simulink model "stateEstimator"  (R2021a)
settings: Solver=ode3  StartTime=0  StopTime=TFinal  FixedStep=Ts  RelTol=1e-3  EnableMultiTasking=on
undefined symbols (not defined in the file): DiscIntNeverNeededParam, Discrete, Estimator, g, init, Sensors, Time, Ts
libraries: simulink x27, ctrlSharedLib x3, sharedtransform x3, sharedutil x1
settings Model: Creator=The MathWorks, Inc.  LastModifiedBy=John
settings SolverCC: AlgebraicLoopSolver=TrustRegion
settings DataIOCC: LimitDataPoints=on  SaveFormat=Array  ReturnWorkspaceOutputs=off
settings OptimizationCC: BlockReduction=off  DefaultParameterBehavior=Inlined  BufferReuse=off  PassReuseOutputArgsThreshold=0
settings DebuggingCC: AlgebraicLoopMsg=none  ParameterPrecisionLossMsg=none  ParameterTunabilityLossMsg=error  UnconnectedInputMsg=none  UnconnectedOutputMsg=none  UnconnectedLineMsg=none  BusObjectLabelMismatch=error  SFUnexpectedBacktrackingDiag=warning  SFNoUnconditionalDefaultTransitionDiag=warning  SFExecutionAtInitializationDiag=none  SFMachineParentedDataDiag=warning  ArithmeticOperatorsInVariantConditions=warning
settings HardwareCC: ProdBitPerPointer=32  ProdBitPerSizeT=32  ProdBitPerPtrDiffT=32  ProdLargestAtomicInteger=Long  ProdWordSize=32  ProdHWDeviceType=ARM Compatible->ARM 9
settings ModelReferenceCC: ModelReferenceNumInstancesAllowed=Single  PropagateSignalLabelsOutOfModel=off
settings SFSimCC: SimUseLocalCustomCode=off  CustomCodeUndefinedFunction=UseInterfaceOnly
settings RTWCC: Description=Generic Real-Time Target  GenCodeOnly=on  GenerateReport=on  RTWUseLocalCustomCode=off  LaunchReport=on
settings CodeAppCC: ForceParamTrailComments=on  MaxIdLength=63  OperatorAnnotations=on  StateflowObjectComments=on  MATLABSourceComments=on
settings GRTTargetCC: TargetLangStandard=C89/C90 (ANSI)
settings ConfigComp: CovMetricSettings=dw  CovSaveCumulativeToWorkspaceVar=on  CovSaveSingleToWorkspaceVar=on  CovExternalEMLEnable=off  CovSFcnEnable=off

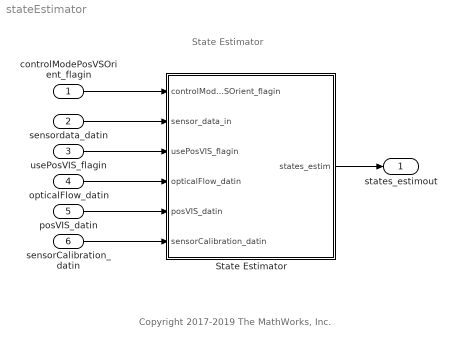
== system stateEstimator ==
  note: State Estimator
  note: Copyright 2017-2019 The MathWorks, Inc.
  controlModePosVSOrient_flagin : Inport  OutDataTypeStr=boolean  SampleTime=Ts
  sensordata_datin : Inport  Port=2  OutDataTypeStr=Bus: sensordata_t  SampleTime=Ts  BusOutputAsStruct=on
  usePosVIS_flagin : Inport  Port=3  OutDataTypeStr=single  SampleTime=Ts
  opticalFlow_datin : Inport  Port=4  OutDataTypeStr=single  SampleTime=Ts
  posVIS_datin : Inport  Port=5  OutDataTypeStr=single  SampleTime=Ts
  sensorCalibration_datin : Inport  Port=6  OutDataTypeStr=single  SampleTime=Ts
  State Estimator : Subsystem
  states_estimout : Outport  OutDataTypeStr=Bus: statesEstim_t  VectorParamsAs1DForOutWhenUnconnected=off  BusOutputAsStruct=on
  wires:
  State Estimator/1(states_estim) -> states_estimout/1
  opticalFlow_datin/1 -> State Estimator/4(opticalFlow_datin)
  controlModePosVSOrient_flagin/1 -> State Estimator/1(controlModePosVSOrient_flagin)
  usePosVIS_flagin/1 -> State Estimator/3(usePosVIS_flagin)
  posVIS_datin/1 -> State Estimator/5(posVIS_datin)
  sensordata_datin/1 -> State Estimator/2(sensor_data_in)
  sensorCalibration_datin/1 -> State Estimator/6(sensorCalibration_datin)

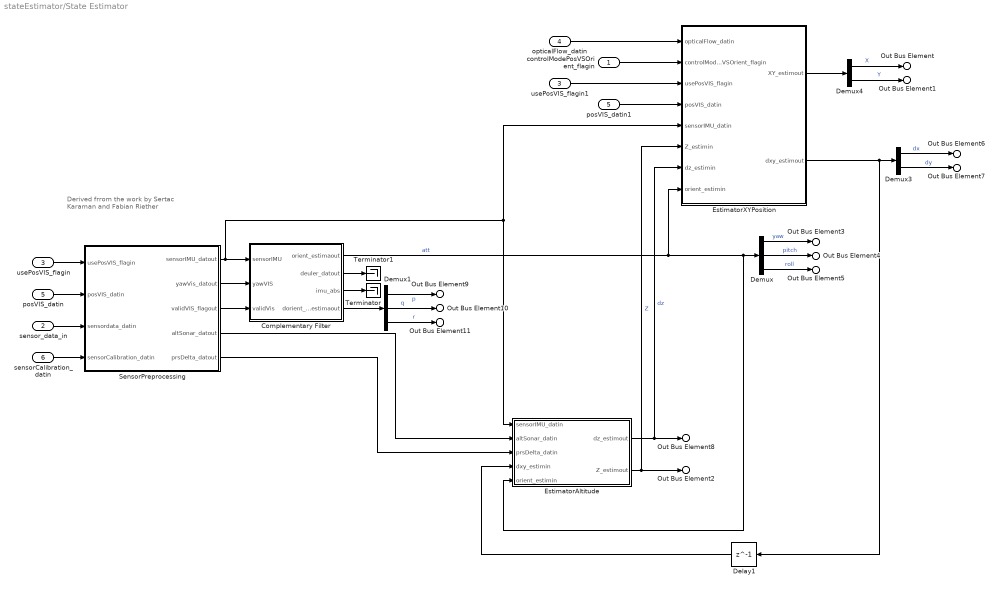
== system stateEstimator/State Estimator ==
  note: Derived frrom the work by Sertac
      | Karaman and Fabian Riether
  controlModePosVSOrient_flagin : Inport  OutDataTypeStr=boolean
  sensor_data_in : Inport  Port=2
  usePosVIS_flagin : Inport  Port=3
  opticalFlow_datin : Inport  Port=4
  posVIS_datin : Inport  Port=5
  sensorCalibration_datin : Inport  Port=6
  Complementary Filter : Subsystem
  Delay1 : Delay  DelayLength=1  InitialCondition=0
  Demux : Demux  Outputs=3
  Demux1 : Demux  Outputs=3
  Demux3 : Demux  Outputs=2
  Demux4 : Demux  Outputs=2
  EstimatorAltitude : Subsystem
  EstimatorXYPosition : Subsystem
  SensorPreprocessing : Subsystem
  Terminator : Terminator
  Terminator1 : Terminator
  posVIS_datin1 : InportShadow  Port=5
  usePosVIS_flagin1 : InportShadow  Port=3
  Out Bus Element : Outport  VectorParamsAs1DForOutWhenUnconnected=off  PortName=states_estim  Element=X
  Out Bus Element1 : Outport  VectorParamsAs1DForOutWhenUnconnected=off  PortName=states_estim  Element=Y
  Out Bus Element2 : Outport  VectorParamsAs1DForOutWhenUnconnected=off  PortName=states_estim  Element=Z
  Out Bus Element3 : Outport  VectorParamsAs1DForOutWhenUnconnected=off  PortName=states_estim  Element=yaw
  Out Bus Element4 : Outport  VectorParamsAs1DForOutWhenUnconnected=off  PortName=states_estim  Element=pitch
  Out Bus Element5 : Outport  VectorParamsAs1DForOutWhenUnconnected=off  PortName=states_estim  Element=roll
  Out Bus Element6 : Outport  VectorParamsAs1DForOutWhenUnconnected=off  PortName=states_estim  Element=dx
  Out Bus Element7 : Outport  VectorParamsAs1DForOutWhenUnconnected=off  PortName=states_estim  Element=dy
  Out Bus Element8 : Outport  VectorParamsAs1DForOutWhenUnconnected=off  PortName=states_estim  Element=dz
  Out Bus Element9 : Outport  VectorParamsAs1DForOutWhenUnconnected=off  PortName=states_estim  Element=p
  Out Bus Element10 : Outport  VectorParamsAs1DForOutWhenUnconnected=off  PortName=states_estim  Element=q
  Out Bus Element11 : Outport  VectorParamsAs1DForOutWhenUnconnected=off  PortName=states_estim  Element=r
  wires:
  EstimatorXYPosition/2(dxy_estimout) -> Delay1/1, Demux3/1
  posVIS_datin/1 -> SensorPreprocessing/2(posVIS_datin)
  Demux1/3 -> Out Bus Element11/1  "r"
  Demux/3 -> Out Bus Element5/1  "roll"
  Demux4/2 -> Out Bus Element1/1  "Y"
  EstimatorXYPosition/1(XY_estimout) -> Demux4/1
  Complementary Filter/2(deuler_datout) -> Terminator1/1
  Complementary Filter/4(dorient_estimaout) -> Demux1/1
  SensorPreprocessing/3(validVIS_flagout) -> Complementary Filter/3(validVis)
  sensor_data_in/1 -> SensorPreprocessing/3(sensordata_datin)
  opticalFlow_datin/1 -> EstimatorXYPosition/1(opticalFlow_datin)
  Demux4/1 -> Out Bus Element/1  "X"
  SensorPreprocessing/1(sensorIMU_datout) -> Complementary Filter/1(sensorIMU), EstimatorAltitude/1(sensorIMU_datin), EstimatorXYPosition/5(sensorIMU_datin)
  SensorPreprocessing/5(prsDelta_datout) -> EstimatorAltitude/3(prsDelta_datin)
  Demux3/2 -> Out Bus Element7/1  "dy"
  SensorPreprocessing/2(yawVis_datout) -> Complementary Filter/2(yawVIS)
  SensorPreprocessing/4(altSonar_datout) -> EstimatorAltitude/2(altSonar_datin)
  usePosVIS_flagin/1 -> SensorPreprocessing/1(usePosVIS_flagin)
  EstimatorAltitude/1(dz_estimout) -> Out Bus Element8/1, EstimatorXYPosition/7(dz_estimin)  "dz"
  EstimatorAltitude/2(Z_estimout) -> Out Bus Element2/1, EstimatorXYPosition/6(Z_estimin)  "Z"
  Demux1/1 -> Out Bus Element9/1  "p"
  Demux3/1 -> Out Bus Element6/1  "dx"
  Complementary Filter/3(imu_abs) -> Terminator/1
  Demux/2 -> Out Bus Element4/1  "pitch"
  controlModePosVSOrient_flagin/1 -> EstimatorXYPosition/2(controlModePosVSOrient_flagin)
  Complementary Filter/1(orient_estimaout) -> EstimatorAltitude/5(orient_estimin), Demux/1, EstimatorXYPosition/8(orient_estimin)  "att"
  Demux/1 -> Out Bus Element3/1  "yaw"
  Delay1/1 -> EstimatorAltitude/4(dxy_estimin)
  Demux1/2 -> Out Bus Element10/1  "q"
  usePosVIS_flagin1/1 -> EstimatorXYPosition/3(usePosVIS_flagin)
  posVIS_datin1/1 -> EstimatorXYPosition/4(posVIS_datin)
  sensorCalibration_datin/1 -> SensorPreprocessing/4(sensorCalibration_datin)

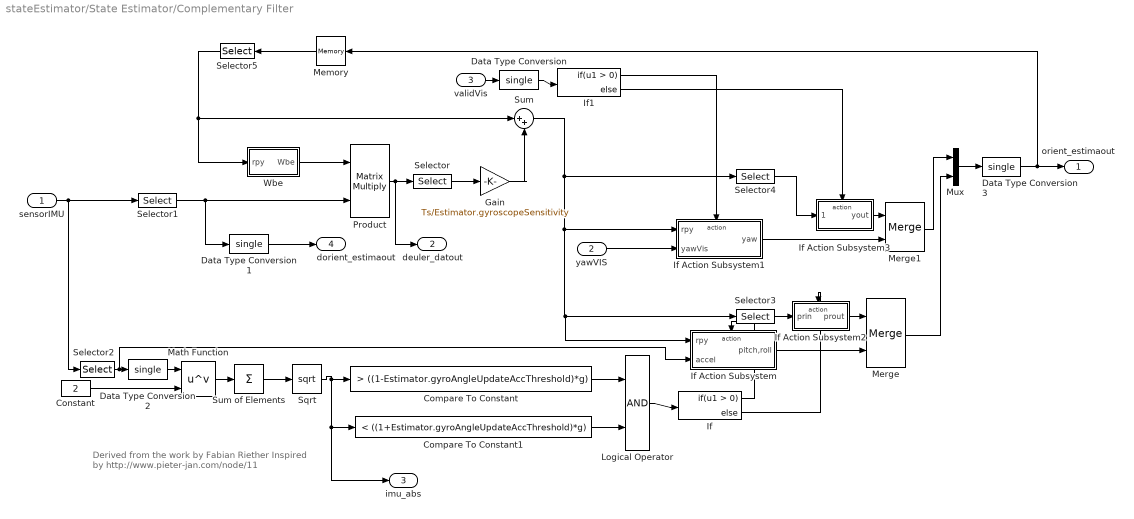
== system stateEstimator/State Estimator/Complementary Filter ==
  note: Derived from the work by Fabian Riether
      | Inspired by http://www.pieter-jan.com/node/11
  sensorIMU : Inport  OutDataTypeStr=single
  yawVIS : Inport  Port=2
  validVis : Inport  Port=3
  Compare To Constant : simulink/Logic and Bit Operations/Compare To Constant  relop=>  const=((1-Estimator.gyroAngleUpdateAccThreshold)*g)  OutDataTypeStr=boolean
  Compare To Constant1 : simulink/Logic and Bit Operations/Compare To Constant  relop=<  const=((1+Estimator.gyroAngleUpdateAccThreshold)*g)  OutDataTypeStr=boolean
  Constant : Constant  Value=2  OutDataTypeStr=single
  Data Type Conversion{,1..3} (4 alike) : DataTypeConversion  OutDataTypeStr=single
  Gain : Gain  Gain=Ts/Estimator.gyroscopeSensitivity
  If : If
  If Action Subsystem : Subsystem  TreatAsAtomicUnit=on
  If Action Subsystem1 : Subsystem  TreatAsAtomicUnit=on
  If Action Subsystem2 : Subsystem  TreatAsAtomicUnit=on
  If Action Subsystem3 : Subsystem  TreatAsAtomicUnit=on
  If1 : If
  Logical Operator : Logic  AllPortsSameDT=off  OutDataTypeStr=fixdt(1,16)
  Math Function : Math  Operator=pow  SignedPower=on  SaturateOnIntegerOverflow=on
  Memory : Memory  InitialCondition=single(Estimator.complementaryFilterInit)  InheritSampleTime=on
  Merge : Merge
  Merge1 : Merge
  Mux : Mux  Inputs=2
  Product : Product  Multiplication=Matrix(*)
  Selector : Selector  InputPortWidth=3  IndexOptions=Index vector (dialog)  Indices=[3 2 1]  OutputSizes=1
  Selector1 : Selector  InputPortWidth=6  IndexOptions=Index vector (dialog)  Indices=[4 5 6]  OutputSizes=1
  Selector2 : Selector  InputPortWidth=6  IndexOptions=Index vector (dialog)  Indices=[1 2 3]  OutputSizes=1
  Selector3 : Selector  InputPortWidth=3  IndexOptions=Index vector (dialog)  Indices=[2 1]  OutputSizes=1
  Selector4 : Selector  InputPortWidth=3  IndexOptions=Index vector (dialog)  Indices=[3]  OutputSizes=1
  Selector5 : Selector  InputPortWidth=3  IndexOptions=Index vector (dialog)  Indices=[3 2 1]  OutputSizes=1
  Sqrt : Sqrt  SaturateOnIntegerOverflow=on
  Sum : Sum  Inputs=|++
  Sum of Elements : Sum  Inputs=+
  Wbe : Subsystem
  orient_estimaout : Outport  VectorParamsAs1DForOutWhenUnconnected=off
  deuler_datout : Outport  Port=2  VectorParamsAs1DForOutWhenUnconnected=off
  imu_abs : Outport  Port=3  OutDataTypeStr=single  VectorParamsAs1DForOutWhenUnconnected=off
  dorient_estimaout : Outport  Port=4  VectorParamsAs1DForOutWhenUnconnected=off
  wires:
  sensorIMU/1 -> Selector1/1, Selector2/1
  Product/1 -> deuler_datout/1, Selector/1
  Wbe/1(Wbe) -> Product/1
  Selector/1 -> Gain/1
  Gain/1 -> Sum/2
  Memory/1 -> Selector5/1
  Sum of Elements/1 -> Sqrt/1
  Math Function/1 -> Sum of Elements/1
  Constant/1 -> Math Function/2
  Selector2/1 -> If Action Subsystem/2(accel), Data Type Conversion2/1
  Sqrt/1 -> imu_abs/1, Compare To Constant1/1, Compare To Constant/1
  Compare To Constant/1 -> Logical Operator/1
  Compare To Constant1/1 -> Logical Operator/2
  If Action Subsystem/1(pitch,roll) -> Merge/2
  Sum/1 -> If Action Subsystem1/1(rpy), If Action Subsystem/1(rpy), Selector3/1, Selector4/1
  Selector3/1 -> If Action Subsystem2/1(prin)
  yawVIS/1 -> If Action Subsystem1/2(yawVis)
  Selector4/1 -> If Action Subsystem3/1(yawin)
  If Action Subsystem1/1(yaw) -> Merge1/2
  Merge/1 -> Mux/2
  Mux/1 -> Data Type Conversion3/1
  If Action Subsystem2/1(prout) -> Merge/1
  If/2 -> If Action Subsystem2/Action
  If Action Subsystem3/1(yout) -> Merge1/1
  If1/2 -> If Action Subsystem3/Action
  Logical Operator/1 -> If/1
  If/1 -> If Action Subsystem/Action
  If1/1 -> If Action Subsystem1/Action
  Data Type Conversion/1 -> If1/1
  validVis/1 -> Data Type Conversion/1
  Selector1/1 -> Product/2, Data Type Conversion1/1
  Data Type Conversion2/1 -> Math Function/1
  Data Type Conversion3/1 -> Memory/1, orient_estimaout/1
  Merge1/1 -> Mux/1
  Selector5/1 -> Sum/1, Wbe/1(rpy)
  Data Type Conversion1/1 -> dorient_estimaout/1

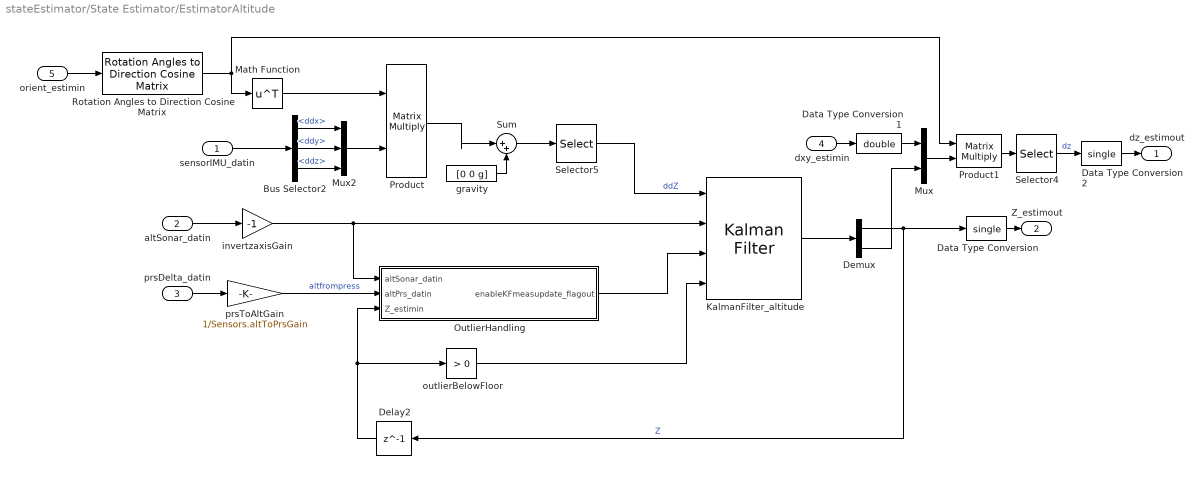
== system stateEstimator/State Estimator/EstimatorAltitude ==
  sensorIMU_datin : Inport
  altSonar_datin : Inport  Port=2
  prsDelta_datin : Inport  Port=3
  dxy_estimin : Inport  Port=4
  orient_estimin : Inport  Port=5
  Bus Selector2 : BusSelector  OutputSignals=ddx,ddy,ddz
  Data Type Conversion : DataTypeConversion  OutDataTypeStr=single  SaturateOnIntegerOverflow=on
  Data Type Conversion1 : DataTypeConversion  OutDataTypeStr=double  SaturateOnIntegerOverflow=on
  Data Type Conversion2 : DataTypeConversion  OutDataTypeStr=single  SaturateOnIntegerOverflow=on
  Delay2 : Delay  DelayLength=1  InitialCondition=0
  Demux : Demux  Outputs=2
  KalmanFilter_altitude : ctrlSharedLib/Kalman Filter  TimeDomain=Discrete-Time  UseCurrentEstimator=on  ModelSource=Individual A, B, C, D matrices  ModelSourceVariable=sys  A=[1 Ts; 0 1]  B=[0;Ts]  C=[1 0]  D=[0]  NumberOfStates=2  NumberOfInputs=2  NumberOfOutputs=2  InitialEstimateSource=Dialog  X0=[init.posNED(3) 0]  P0=10  UseK=off  UseGH=on  NumberOfProcessNoiseInputs=2  G=Estimator.alt.kf.G  TimeInvariantG=on  H=Estimator.alt.kf.H  TimeInvariantH=on  Q=Estimator.alt.kf.Q  TimeInvariantQ=on  R=Estimator.alt.kf.R  TimeInvariantR=on  N=Estimator.alt.kf.N  TimeInvariantN=on  AddInputPort=on  AddEnablePort=on  ExternalReset=Level hold  OutputEstimatedY=off  OutputP=off  Ts=-1
  Math Function : Math  Operator=transpose  SignedPower=on  SaturateOnIntegerOverflow=on
  Mux : Mux  Inputs=2
  Mux2 : Mux  Inputs=3
  OutlierHandling : Subsystem
  Product : Product  Multiplication=Matrix(*)
  Product1 : Product  Multiplication=Matrix(*)
  Rotation Angles to Direction Cosine Matrix : sharedtransform/Rotation Angles to Direction Cosine Matrix  rotationOrder=ZYX  aMode=aMode
      settings: SourceProductBaseCode=AE,PW,DR,MT,UV,VE
  Selector4 : Selector  InputPortWidth=3  IndexOptions=Index vector (dialog)  Indices=[3]  OutputSizes=1
  Selector5 : Selector  InputPortWidth=3  IndexOptions=Index vector (dialog)  Indices=[3]  OutputSizes=1
  Sum : Sum  Inputs=|++
  gravity : Constant  Value=[0 0 g]
  invertzaxisGain : Gain  Gain=-1  ParamDataTypeStr=single  OutDataTypeStr=double
  outlierBelowFloor : simulink/Logic and Bit Operations/Compare To Constant  relop=>  const=0  OutDataTypeStr=boolean
  prsToAltGain : Gain  Gain=1/Sensors.altToPrsGain
  dz_estimout : Outport  VectorParamsAs1DForOutWhenUnconnected=off
  Z_estimout : Outport  Port=2  VectorParamsAs1DForOutWhenUnconnected=off
  wires:
  Mux2/1 -> Product/2
  sensorIMU_datin/1 -> Bus Selector2/1
  Bus Selector2/3 -> Mux2/3  "<ddz>"
  Bus Selector2/2 -> Mux2/2  "<ddy>"
  Bus Selector2/1 -> Mux2/1  "<ddx>"
  Product1/1 -> Selector4/1
  dxy_estimin/1 -> Data Type Conversion1/1
  Delay2/1 -> OutlierHandling/3(Z_estimin), outlierBelowFloor/1
  prsToAltGain/1 -> OutlierHandling/2(altPrs_datin)  "altfrompress"
  prsDelta_datin/1 -> prsToAltGain/1
  outlierBelowFloor/1 -> KalmanFilter_altitude/4
  Demux/2 -> Mux/2
  Selector4/1 -> Data Type Conversion2/1  "dz"
  Demux/1 -> Data Type Conversion/1, Delay2/1  "Z"
  Selector5/1 -> KalmanFilter_altitude/1  "ddZ"
  Mux/1 -> Product1/2
  KalmanFilter_altitude/1 -> Demux/1
  Sum/1 -> Selector5/1
  gravity/1 -> Sum/2
  Product/1 -> Sum/1
  altSonar_datin/1 -> invertzaxisGain/1
  orient_estimin/1 -> Rotation Angles to Direction Cosine Matrix/1
  Data Type Conversion/1 -> Z_estimout/1
  Data Type Conversion1/1 -> Mux/1
  Math Function/1 -> Product/1
  invertzaxisGain/1 -> KalmanFilter_altitude/2, OutlierHandling/1(altSonar_datin)
  Data Type Conversion2/1 -> dz_estimout/1
  OutlierHandling/1(enableKFmeasupdate_flagout) -> KalmanFilter_altitude/3
  Rotation Angles to Direction Cosine Matrix/1 -> Math Function/1, Product1/1

== system stateEstimator/State Estimator/EstimatorXYPosition ==
  opticalFlow_datin : Inport
  controlModePosVSOrient_flagin : Inport  Port=2
  usePosVIS_flagin : Inport  Port=3
  posVIS_datin : Inport  Port=4
  sensorIMU_datin : Inport  Port=5
  Z_estimin : Inport  Port=6
  dz_estimin : Inport  Port=7
  orient_estimin : Inport  Port=8
  EstimatorVelocity : Subsystem
  EstimatorXYPosition : Subsystem
  XY_estimout : Outport  VectorParamsAs1DForOutWhenUnconnected=off
  dxy_estimout : Outport  Port=2  VectorParamsAs1DForOutWhenUnconnected=off
  wires:
  EstimatorXYPosition/1(XY_estimout) -> XY_estimout/1
  usePosVIS_flagin/1 -> EstimatorXYPosition/6(usePosVIS_flagin)
  posVIS_datin/1 -> EstimatorXYPosition/5(posVIS_datin)
  dz_estimin/1 -> EstimatorXYPosition/4(dz_estimin)
  controlModePosVSOrient_flagin/1 -> EstimatorXYPosition/3(controlModePosVSOrient_flagin)
  Z_estimin/1 -> EstimatorVelocity/2(Z_estimin)
  sensorIMU_datin/1 -> EstimatorVelocity/3(sensorIMU_datin)
  opticalFlow_datin/1 -> EstimatorVelocity/1(opticalFlow_datin)
  EstimatorVelocity/1(dxy_estimout) -> dxy_estimout/1, EstimatorXYPosition/1(dxy_estimin)
  orient_estimin/1 -> EstimatorXYPosition/2(orient_estimin), EstimatorVelocity/4(orient_estimin)

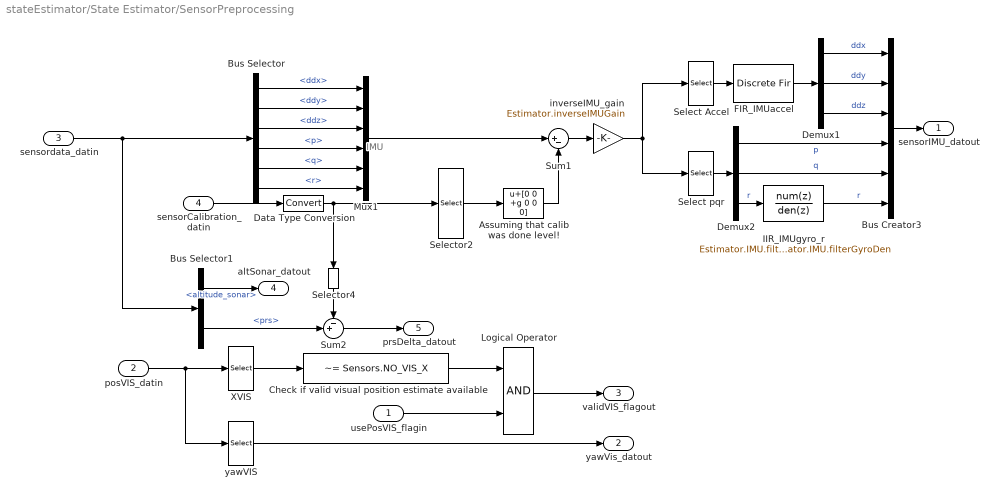
== system stateEstimator/State Estimator/SensorPreprocessing ==
  note: IMU
  usePosVIS_flagin : Inport
  posVIS_datin : Inport  Port=2
  sensordata_datin : Inport  Port=3
  sensorCalibration_datin : Inport  Port=4
  Assuming that calib was done level! : Bias  Bias=[0 0 +g 0 0 0]
  Bus Creator3 : BusCreator  Inputs=6
  Bus Selector : BusSelector  OutputSignals=ddx,ddy,ddz,p,q,r
  Bus Selector1 : BusSelector  OutputSignals=altitude_sonar,prs
  Check if valid visual position estimate available : simulink/Logic and Bit Operations/Compare To Constant  relop=~=  const=Sensors.NO_VIS_X  OutDataTypeStr=boolean
  Data Type Conversion : DataTypeConversion
  Demux1 : Demux  Outputs=3
  Demux2 : Demux  Outputs=3
  FIR_IMUaccel : DiscreteFir  Coefficients=Estimator.IMU.filterAccel.Coefficients
  IIR_IMUgyro_r : DiscreteFilter  Numerator=Estimator.IMU.filterGyroNum  Denominator=Estimator.IMU.filterGyroDen
  Logical Operator : Logic  AllPortsSameDT=off  OutDataTypeStr=boolean
  Mux1 : Mux  Inputs=6
  Select Accel : Selector  InputPortWidth=6  IndexOptions=Index vector (dialog)  Indices=[1 2 3]  OutputSizes=1
  Select pqr : Selector  InputPortWidth=6  IndexOptions=Index vector (dialog)  Indices=[4 5 6]  OutputSizes=1
  Selector2 : Selector  InputPortWidth=8  IndexOptions=Index vector (dialog)  Indices=[1:6]  OutputSizes=1
  Selector4 : Selector  InputPortWidth=8  IndexOptions=Index vector (dialog)  Indices=[7]  OutputSizes=1
  Sum1 : Sum  Inputs=|+-
  Sum2 : Sum  Inputs=-+|
  XVIS : Selector  InputPortWidth=4  IndexOptions=Index vector (dialog)  Indices=1  OutputSizes=1
  inverseIMU_gain : Gain  Gain=Estimator.inverseIMUGain  ParamDataTypeStr=single  OutDataTypeStr=single
  yawVIS : Selector  InputPortWidth=4  IndexOptions=Index vector (dialog)  Indices=4  OutputSizes=1
  sensorIMU_datout : Outport  VectorParamsAs1DForOutWhenUnconnected=off
  yawVis_datout : Outport  Port=2  VectorParamsAs1DForOutWhenUnconnected=off
  validVIS_flagout : Outport  Port=3  VectorParamsAs1DForOutWhenUnconnected=off
  altSonar_datout : Outport  Port=4  VectorParamsAs1DForOutWhenUnconnected=off
  prsDelta_datout : Outport  Port=5  VectorParamsAs1DForOutWhenUnconnected=off
  wires:
  Select pqr/1 -> Demux2/1
  Assuming that calib was done level!/1 -> Sum1/2
  usePosVIS_flagin/1 -> Logical Operator/2
  Check if valid visual position estimate available/1 -> Logical Operator/1
  Logical Operator/1 -> validVIS_flagout/1
  yawVIS/1 -> yawVis_datout/1
  XVIS/1 -> Check if valid visual position estimate available/1
  Mux1/1 -> Sum1/1
  Sum2/1 -> prsDelta_datout/1
  Bus Selector1/2 -> Sum2/2  "<prs>"
  Selector4/1 -> Sum2/1
  Bus Selector1/1 -> altSonar_datout/1  "<altitude_sonar>"
  sensordata_datin/1 -> Bus Selector1/1, Bus Selector/1
  Bus Selector/6 -> Mux1/6  "<r>"
  Bus Selector/5 -> Mux1/5  "<q>"
  Bus Selector/4 -> Mux1/4  "<p>"
  Bus Selector/3 -> Mux1/3  "<ddz>"
  Bus Selector/2 -> Mux1/2  "<ddy>"
  Bus Selector/1 -> Mux1/1  "<ddx>"
  sensorCalibration_datin/1 -> Data Type Conversion/1
  IIR_IMUgyro_r/1 -> Bus Creator3/6  "r"
  Demux2/3 -> IIR_IMUgyro_r/1  "r"
  FIR_IMUaccel/1 -> Demux1/1
  Select Accel/1 -> FIR_IMUaccel/1
  inverseIMU_gain/1 -> Select Accel/1, Select pqr/1
  Demux2/2 -> Bus Creator3/5  "q"
  Demux2/1 -> Bus Creator3/4  "p"
  Selector2/1 -> Assuming that calib was done level!/1
  Sum1/1 -> inverseIMU_gain/1
  Demux1/3 -> Bus Creator3/3  "ddz"
  Demux1/2 -> Bus Creator3/2  "ddy"
  Demux1/1 -> Bus Creator3/1  "ddx"
  Bus Creator3/1 -> sensorIMU_datout/1
  posVIS_datin/1 -> XVIS/1, yawVIS/1
  Data Type Conversion/1 -> Selector2/1, Selector4/1

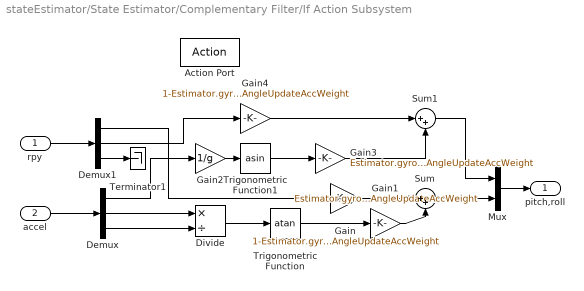
== system stateEstimator/State Estimator/Complementary Filter/If Action Subsystem ==
  rpy : Inport
  accel : Inport  Port=2
  Action Port : ActionPort  ActionPortLabel=if(u1 > 0)
  Demux : Demux  Outputs=3
  Demux1 : Demux  Outputs=3
  Divide : Product  Inputs=*/
  Gain : Gain  Gain=1-Estimator.gyroAngleUpdateAccWeight
  Gain1 : Gain  Gain=Estimator.gyroAngleUpdateAccWeight
  Gain2 : Gain  Gain=1/g
  Gain3 : Gain  Gain=Estimator.gyroAngleUpdateAccWeight
  Gain4 : Gain  Gain=1-Estimator.gyroAngleUpdateAccWeight
  Mux : Mux  Inputs=2
  Sum : Sum  Inputs=|++
  Sum1 : Sum  Inputs=|++
  Terminator1 : Terminator
  Trigonometric Function : Trigonometry  Operator=atan
  Trigonometric Function1 : Trigonometry  Operator=asin
  pitch,roll : Outport  VectorParamsAs1DForOutWhenUnconnected=off
  wires:
  accel/1 -> Demux/1
  Demux/2 -> Divide/1
  Demux/3 -> Divide/2
  Divide/1 -> Trigonometric Function/1
  Gain/1 -> Sum/1
  Trigonometric Function/1 -> Gain1/1
  Mux/1 -> pitch,roll/1
  Gain2/1 -> Trigonometric Function1/1
  Trigonometric Function1/1 -> Gain3/1
  Gain4/1 -> Sum1/1
  Gain3/1 -> Sum1/2
  Sum1/1 -> Mux/1
  Sum/1 -> Mux/2
  rpy/1 -> Demux1/1
  Demux1/1 -> Gain/1
  Demux1/2 -> Gain4/1
  Demux/1 -> Gain2/1
  Demux1/3 -> Terminator1/1
  Gain1/1 -> Sum/2

== system stateEstimator/State Estimator/Complementary Filter/If Action Subsystem1 ==
  rpy : Inport
  yawVis : Inport  Port=2
  Action Port : ActionPort  ActionPortLabel=if(u1 > 0)
  Gain : Gain  Gain=1-Estimator.gyroAngleUpdateVisWeight
  Gain1 : Gain  Gain=Estimator.gyroAngleUpdateVisWeight
  Selector4 : Selector  InputPortWidth=3  IndexOptions=Index vector (dialog)  Indices=[3]  OutputSizes=1
  Sum : Sum  Inputs=|++
  yaw : Outport  VectorParamsAs1DForOutWhenUnconnected=off
  wires:
  rpy/1 -> Selector4/1
  Selector4/1 -> Gain/1
  yawVis/1 -> Gain1/1
  Gain/1 -> Sum/1
  Gain1/1 -> Sum/2
  Sum/1 -> yaw/1

== system stateEstimator/State Estimator/Complementary Filter/If Action Subsystem2 ==
  prin : Inport
  Action Port : ActionPort  ActionPortLabel=else
  prout : Outport  VectorParamsAs1DForOutWhenUnconnected=off
  wires:
  prin/1 -> prout/1

== system stateEstimator/State Estimator/Complementary Filter/If Action Subsystem3 ==
  yawin : Inport
  Action Port : ActionPort  ActionPortLabel=else
  yout : Outport  VectorParamsAs1DForOutWhenUnconnected=off
  wires:
  yawin/1 -> yout/1

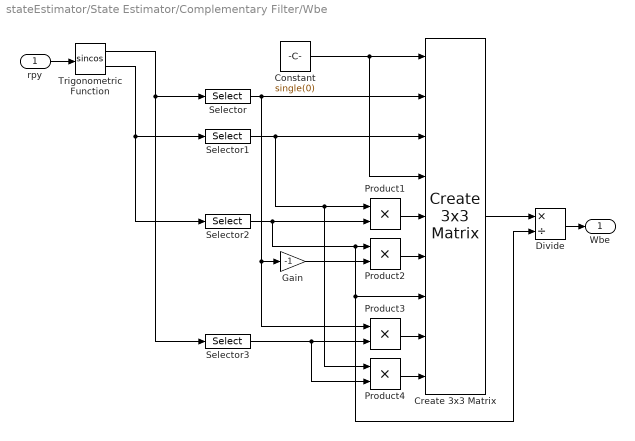
== system stateEstimator/State Estimator/Complementary Filter/Wbe ==
  rpy : Inport  OutDataTypeStr=single
  Constant : Constant  Value=single(0)
  Create 3x3 Matrix : sharedutil/Create 3x3 Matrix  aMode=aMode
      settings: SourceProductBaseCode=AE,PW,DR,MT,UV,VE
  Divide : Product  Inputs=*/
  Gain : Gain  Gain=-1
  Product{1..4} (4 alike) : Product
  Selector : Selector  InputPortWidth=3  IndexOptions=Index vector (dialog)  Indices=[1]  OutputSizes=1
  Selector1 : Selector  InputPortWidth=3  IndexOptions=Index vector (dialog)  Indices=[1]  OutputSizes=1
  Selector2 : Selector  InputPortWidth=3  IndexOptions=Index vector (dialog)  Indices=[2]  OutputSizes=1
  Selector3 : Selector  InputPortWidth=3  IndexOptions=Index vector (dialog)  Indices=[2]  OutputSizes=1
  Trigonometric Function : Trigonometry  Operator=sincos
  Wbe : Outport  VectorParamsAs1DForOutWhenUnconnected=off
  wires:
  Create 3x3 Matrix/1 -> Divide/1
  Product3/1 -> Create 3x3 Matrix/8
  Trigonometric Function/2 -> Selector1/1, Selector2/1
  Selector3/1 -> Product4/2, Product3/2
  Selector1/1 -> Product4/1, Product1/1, Create 3x3 Matrix/3
  Trigonometric Function/1 -> Selector3/1, Selector/1
  Product1/1 -> Create 3x3 Matrix/5
  Product2/1 -> Create 3x3 Matrix/6
  Selector2/1 -> Divide/2, Create 3x3 Matrix/7, Product2/1, Product1/2
  Gain/1 -> Product2/2
  Product4/1 -> Create 3x3 Matrix/9
  Constant/1 -> Create 3x3 Matrix/4, Create 3x3 Matrix/1
  Divide/1 -> Wbe/1
  rpy/1 -> Trigonometric Function/1
  Selector/1 -> Product3/1, Gain/1, Create 3x3 Matrix/2

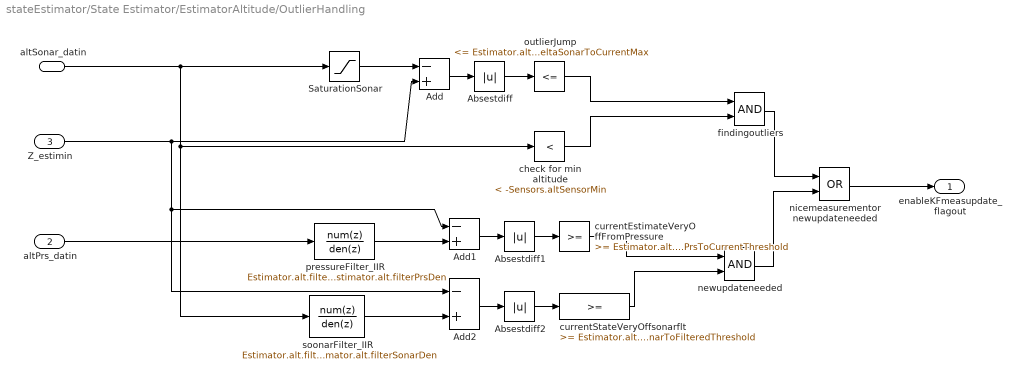
== system stateEstimator/State Estimator/EstimatorAltitude/OutlierHandling ==
  altSonar_datin : Inport
  altPrs_datin : Inport  Port=2
  Z_estimin : Inport  Port=3
  Absestdiff : Abs
  Absestdiff1 : Abs
  Absestdiff2 : Abs
  Add : Sum  Inputs=-+
  Add1 : Sum  Inputs=-+
  Add2 : Sum  Inputs=-+
  SaturationSonar : Saturate  UpperLimit=-Sensors.altSensorMin  LowerLimit=-inf
  check for min altitude : simulink/Logic and Bit Operations/Compare To Constant  relop=<  const=-Sensors.altSensorMin  OutDataTypeStr=boolean
  currentEstimateVeryOffFromPressure : simulink/Logic and Bit Operations/Compare To Constant  relop=>=  const=Estimator.alt.deltaPrsToCurrentThreshold  OutDataTypeStr=boolean
  currentStateVeryOffsonarflt : simulink/Logic and Bit Operations/Compare To Constant  relop=>=  const=Estimator.alt.deltaSonarToFilteredThreshold  OutDataTypeStr=boolean
  findingoutliers : Logic  AllPortsSameDT=off  OutDataTypeStr=boolean
  newupdateneeded : Logic  AllPortsSameDT=off  OutDataTypeStr=boolean
  nicemeasurementor newupdateneeded : Logic  Operator=OR  AllPortsSameDT=off  OutDataTypeStr=boolean
  outlierJump : simulink/Logic and Bit Operations/Compare To Constant  relop=<=  const=Estimator.alt.deltaSonarToCurrentMax  OutDataTypeStr=boolean
  pressureFilter_IIR : DiscreteFilter  Numerator=Estimator.alt.filterPrsNum  Denominator=Estimator.alt.filterPrsDen
  soonarFilter_IIR : DiscreteFilter  Numerator=Estimator.alt.filterSonarNum  Denominator=Estimator.alt.filterSonarDen
  enableKFmeasupdate_flagout : Outport  VectorParamsAs1DForOutWhenUnconnected=off
  wires:
  Add1/1 -> Absestdiff1/1
  nicemeasurementor newupdateneeded/1 -> enableKFmeasupdate_flagout/1
  findingoutliers/1 -> nicemeasurementor newupdateneeded/1
  check for min altitude/1 -> findingoutliers/2
  outlierJump/1 -> findingoutliers/1
  SaturationSonar/1 -> Add/1
  Absestdiff/1 -> outlierJump/1
  Add/1 -> Absestdiff/1
  newupdateneeded/1 -> nicemeasurementor newupdateneeded/2
  Absestdiff2/1 -> currentStateVeryOffsonarflt/1
  altSonar_datin/1 -> SaturationSonar/1, soonarFilter_IIR/1, check for min altitude/1
  currentEstimateVeryOffFromPressure/1 -> newupdateneeded/1
  Z_estimin/1 -> Add1/1, Add2/1, Add/2
  Add2/1 -> Absestdiff2/1
  currentStateVeryOffsonarflt/1 -> newupdateneeded/2
  pressureFilter_IIR/1 -> Add1/2
  altPrs_datin/1 -> pressureFilter_IIR/1
  soonarFilter_IIR/1 -> Add2/2
  Absestdiff1/1 -> currentEstimateVeryOffFromPressure/1

== system stateEstimator/State Estimator/EstimatorXYPosition/EstimatorVelocity ==
  opticalFlow_datin : Inport
  Z_estimin : Inport  Port=2  SampleTime=Ts
  sensorIMU_datin : Inport  Port=3
  orient_estimin : Inport  Port=4
  AccelerationHandling : Subsystem
  DataHandling : Subsystem
  Delay : Delay  DelayLength=1  InitialCondition=0
  KalmanFilter_dxdy : ctrlSharedLib/Kalman Filter  TimeDomain=Discrete-Time  UseCurrentEstimator=on  ModelSource=Individual A, B, C, D matrices  ModelSourceVariable=ss(0.95,1,1,0,1)  A=eye(2)  B=Ts*eye(2)  C=eye(2)  D=0  NumberOfStates=1  NumberOfInputs=1  NumberOfOutputs=1  InitialEstimateSource=Dialog  X0=0  P0=10  UseK=off  UseGH=on  NumberOfProcessNoiseInputs=1  G=Estimator.pos.kfVelo.G  TimeInvariantG=on  H=Estimator.pos.kfVelo.H  TimeInvariantH=on  Q=Estimator.pos.kfVelo.Q  TimeInvariantQ=on  R=Estimator.pos.kfVelo.R  TimeInvariantR=on  N=Estimator.pos.kfVelo.N  TimeInvariantN=on  AddInputPort=on  AddEnablePort=on  OutputEstimatedY=off  OutputP=off  Ts=-1
  Select dxy : Selector  InputPortWidth=3  IndexOptions=Index vector (dialog)  Indices=[1 2]  OutputSizes=1
  opticalFlowToVelocity_gain : Gain  Gain=Estimator.pos.opticalFlowToVelocityGain
  dxy_estimout : Outport  VectorParamsAs1DForOutWhenUnconnected=off
  wires:
  Delay/1 -> DataHandling/5(dxyOF_datin)
  Z_estimin/1 -> DataHandling/1(Z_estimin), AccelerationHandling/4(Z_estimin)
  KalmanFilter_dxdy/1 -> dxy_estimout/1, Delay/1
  opticalFlowToVelocity_gain/1 -> Select dxy/1
  opticalFlow_datin/1 -> opticalFlowToVelocity_gain/1
  sensorIMU_datin/1 -> AccelerationHandling/2(sensorIMU_datin), DataHandling/3(sensorIMU_datin)
  orient_estimin/1 -> AccelerationHandling/3(orient_estimin), DataHandling/2(orient_estimin)
  Select dxy/1 -> KalmanFilter_dxdy/2, AccelerationHandling/1(dxy_estimin), DataHandling/4(dxy_estimin)
  AccelerationHandling/1(acceleration_world) -> KalmanFilter_dxdy/1
  DataHandling/1(enable_flag) -> KalmanFilter_dxdy/3

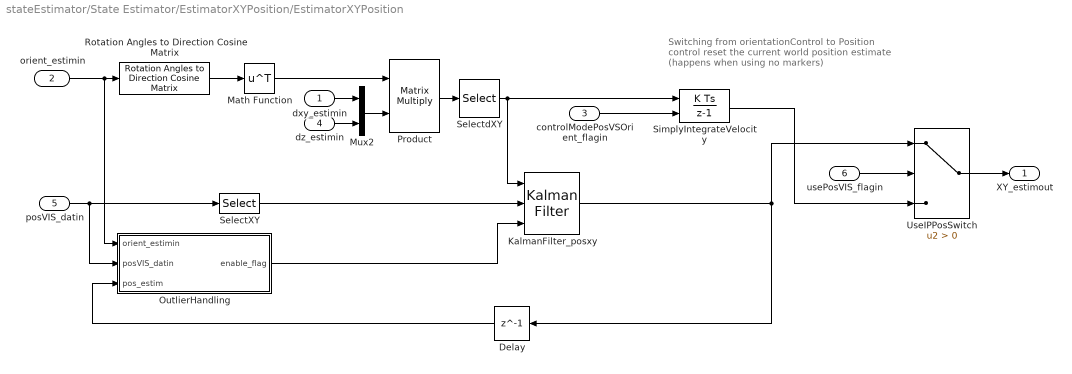
== system stateEstimator/State Estimator/EstimatorXYPosition/EstimatorXYPosition ==
  note: Switching from orientationControl to Position
      | control reset the current world position estimate
      | (happens when using no markers)
  dxy_estimin : Inport
  orient_estimin : Inport  Port=2  SampleTime=Ts
  controlModePosVSOrient_flagin : Inport  Port=3
  dz_estimin : Inport  Port=4
  posVIS_datin : Inport  Port=5
  usePosVIS_flagin : Inport  Port=6
  Delay : Delay  DelayLength=1  InitialCondition=0
  KalmanFilter_posxy : ctrlSharedLib/Kalman Filter  TimeDomain=Discrete-Time  UseCurrentEstimator=on  ModelSource=Individual A, B, C, D matrices  ModelSourceVariable=ss(0.95,1,1,0,1)  A=eye(2)  B=Ts*eye(2)  C=eye(2)  D=0  NumberOfStates=1  NumberOfInputs=1  NumberOfOutputs=1  InitialEstimateSource=Dialog  X0=[.1 0]  P0=10  UseK=off  UseGH=on  NumberOfProcessNoiseInputs=1  G=Estimator.pos.kfPos.G  TimeInvariantG=on  H=Estimator.pos.kfPos.H  TimeInvariantH=on  Q=Estimator.pos.kfPos.Q  TimeInvariantQ=on  R=Estimator.pos.kfPos.R  TimeInvariantR=on  N=Estimator.pos.kfPos.N  TimeInvariantN=on  AddInputPort=on  AddEnablePort=on  OutputEstimatedY=off  OutputP=off  Ts=-1
  Math Function : Math  Operator=transpose  SignedPower=on  SaturateOnIntegerOverflow=on
  Mux2 : Mux  Inputs=2
  OutlierHandling : Subsystem
  Product : Product  Multiplication=Matrix(*)
  Rotation Angles to Direction Cosine Matrix : sharedtransform/Rotation Angles to Direction Cosine Matrix  rotationOrder=ZYX  aMode=aMode
      settings: SourceProductBaseCode=AE,PW,DR,MT,UV,VE
  SelectXY : Selector  InputPortWidth=4  IndexOptions=Index vector (dialog)  Indices=[1 2]  OutputSizes=1
  SelectdXY : Selector  InputPortWidth=3  IndexOptions=Index vector (dialog)  Indices=[1 2]  OutputSizes=1
  SimplyIntegrateVelocity : DiscreteIntegrator  ExternalReset=rising  SampleTime=Ts  ICPrevOutput=DiscIntNeverNeededParam  ICPrevScaledInput=DiscIntNeverNeededParam
  UseIPPosSwitch : Switch  Criteria=u2 > Threshold
  XY_estimout : Outport  VectorParamsAs1DForOutWhenUnconnected=off
  wires:
  Delay/1 -> OutlierHandling/3(pos_estim)
  usePosVIS_flagin/1 -> UseIPPosSwitch/2
  UseIPPosSwitch/1 -> XY_estimout/1
  controlModePosVSOrient_flagin/1 -> SimplyIntegrateVelocity/2
  KalmanFilter_posxy/1 -> Delay/1, UseIPPosSwitch/1
  posVIS_datin/1 -> OutlierHandling/2(posVIS_datin), SelectXY/1
  Product/1 -> SelectdXY/1
  Mux2/1 -> Product/2
  dz_estimin/1 -> Mux2/2
  SimplyIntegrateVelocity/1 -> UseIPPosSwitch/3
  dxy_estimin/1 -> Mux2/1
  orient_estimin/1 -> Rotation Angles to Direction Cosine Matrix/1, OutlierHandling/1(orient_estimin)
  Rotation Angles to Direction Cosine Matrix/1 -> Math Function/1
  SelectXY/1 -> KalmanFilter_posxy/2
  OutlierHandling/1(enable_flag) -> KalmanFilter_posxy/3
  SelectdXY/1 -> SimplyIntegrateVelocity/1, KalmanFilter_posxy/1
  Math Function/1 -> Product/1

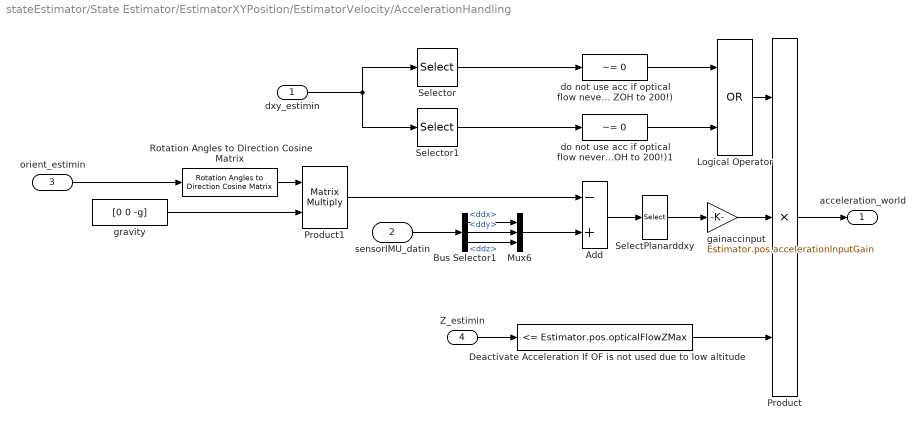
== system stateEstimator/State Estimator/EstimatorXYPosition/EstimatorVelocity/AccelerationHandling ==
  dxy_estimin : Inport
  sensorIMU_datin : Inport  Port=2
  orient_estimin : Inport  Port=3
  Z_estimin : Inport  Port=4
  Add : Sum  Inputs=-+
  Bus Selector1 : BusSelector  OutputSignals=ddx,ddy,ddz
  Deactivate Acceleration If OF is not used due to low altitude : simulink/Logic and Bit Operations/Compare To Constant  relop=<=  const=Estimator.pos.opticalFlowZMax  OutDataTypeStr=boolean
  Logical Operator : Logic  Operator=OR  AllPortsSameDT=off  OutDataTypeStr=boolean
  Mux6 : Mux  Inputs=3
  Product : Product  Inputs=3
  Product1 : Product  Multiplication=Matrix(*)
  Rotation Angles to Direction Cosine Matrix : sharedtransform/Rotation Angles to Direction Cosine Matrix  rotationOrder=ZYX  aMode=aMode
      settings: SourceProductBaseCode=AE,PW,DR,MT,UV,VE
  SelectPlanarddxy : Selector  InputPortWidth=3  IndexOptions=Index vector (dialog)  Indices=[1 2]  OutputSizes=1
  Selector : Selector  InputPortWidth=2  IndexOptions=Index vector (dialog)  Indices=1  OutputSizes=1
  Selector1 : Selector  InputPortWidth=2  IndexOptions=Index vector (dialog)  Indices=2  OutputSizes=1
  do not use acc if optical flow never available (Note OF@60Hz but ZOH to 200!) : simulink/Logic and Bit Operations/Compare To Constant  relop=~=  const=0  OutDataTypeStr=boolean
  do not use acc if optical flow never available (Note OF@60Hz but ZOH to 200!)1 : simulink/Logic and Bit Operations/Compare To Constant  relop=~=  const=0  OutDataTypeStr=boolean
  gainaccinput : Gain  Gain=Estimator.pos.accelerationInputGain  OutDataTypeStr=single
  gravity : Constant  Value=[0 0 -g]
  acceleration_world : Outport  OutDataTypeStr=single  VectorParamsAs1DForOutWhenUnconnected=off
  wires:
  do not use acc if optical flow never available (Note OF@60Hz but ZOH to 200!)1/1 -> Logical Operator/2
  do not use acc if optical flow never available (Note OF@60Hz but ZOH to 200!)/1 -> Logical Operator/1
  Logical Operator/1 -> Product/1
  Selector1/1 -> do not use acc if optical flow never available (Note OF@60Hz but ZOH to 200!)1/1
  Selector/1 -> do not use acc if optical flow never available (Note OF@60Hz but ZOH to 200!)/1
  dxy_estimin/1 -> Selector1/1, Selector/1
  Product/1 -> acceleration_world/1
  Deactivate Acceleration If OF is not used due to low altitude/1 -> Product/3
  Z_estimin/1 -> Deactivate Acceleration If OF is not used due to low altitude/1
  Add/1 -> SelectPlanarddxy/1
  Product1/1 -> Add/1
  gravity/1 -> Product1/2
  gainaccinput/1 -> Product/2
  SelectPlanarddxy/1 -> gainaccinput/1
  Bus Selector1/3 -> Mux6/3  "<ddz>"
  Bus Selector1/1 -> Mux6/1  "<ddx>"
  sensorIMU_datin/1 -> Bus Selector1/1
  Mux6/1 -> Add/2
  Bus Selector1/2 -> Mux6/2  "<ddy>"
  orient_estimin/1 -> Rotation Angles to Direction Cosine Matrix/1
  Rotation Angles to Direction Cosine Matrix/1 -> Product1/1

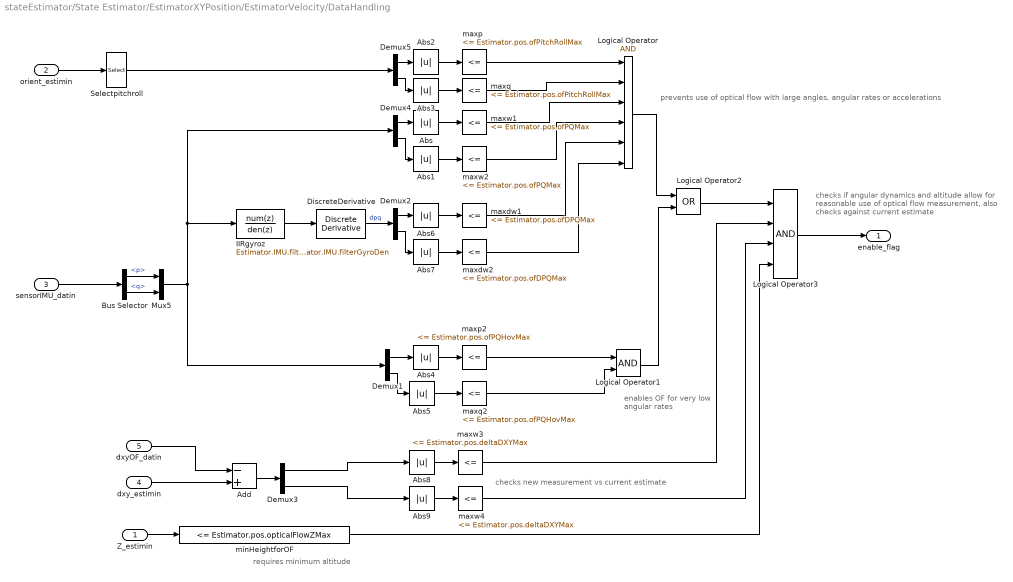
== system stateEstimator/State Estimator/EstimatorXYPosition/EstimatorVelocity/DataHandling ==
  note: prevents use of optical flow with large angles, angular rates or accelerations
  note: enables OF for very
      | low angular rates
  note: checks if angular dynamics and altitude allow for
      | reasonable use of optical flow measurement,
      | also checks against current estimate
  note: checks new measurement vs current estimate
  note: requires minimum altitude
  Z_estimin : Inport
  orient_estimin : Inport  Port=2
  sensorIMU_datin : Inport  Port=3
  dxy_estimin : Inport  Port=4
  dxyOF_datin : Inport  Port=5
  Abs{,1..9} (10 alike) : Abs
  Add : Sum  Inputs=-+
  Bus Selector : BusSelector  OutputSignals=p,q
  Demux{1..5} (5 alike) : Demux  Outputs=2
  DiscreteDerivative : simulink/Discrete/Discrete Derivative  gainval=1.0  ICPrevScaledInput=0.0  OutMin=[]  OutMax=[]  OutDataType=fixdt(1, 16)  OutScaling=2^-10  DoSatur=off
  IIRgyroz : DiscreteFilter  Numerator=Estimator.IMU.filterGyroNum  Denominator=Estimator.IMU.filterGyroDen
  Logical Operator : Logic  Inputs=6  AllPortsSameDT=off  OutDataTypeStr=boolean
  Logical Operator1 : Logic  AllPortsSameDT=off  OutDataTypeStr=boolean
  Logical Operator2 : Logic  Operator=OR  AllPortsSameDT=off  OutDataTypeStr=boolean
  Logical Operator3 : Logic  Inputs=4  AllPortsSameDT=off  OutDataTypeStr=boolean
  Mux5 : Mux  Inputs=2
  Selectpitchroll : Selector  InputPortWidth=3  IndexOptions=Index vector (dialog)  Indices=[2 3]  OutputSizes=1
  maxdw1 : simulink/Logic and Bit Operations/Compare To Constant  relop=<=  const=Estimator.pos.ofDPQMax  OutDataTypeStr=boolean
  maxdw2 : simulink/Logic and Bit Operations/Compare To Constant  relop=<=  const=Estimator.pos.ofDPQMax  OutDataTypeStr=boolean
  maxp : simulink/Logic and Bit Operations/Compare To Constant  relop=<=  const=Estimator.pos.ofPitchRollMax  OutDataTypeStr=boolean
  maxp2 : simulink/Logic and Bit Operations/Compare To Constant  relop=<=  const=Estimator.pos.ofPQHovMax  OutDataTypeStr=boolean
  maxq : simulink/Logic and Bit Operations/Compare To Constant  relop=<=  const=Estimator.pos.ofPitchRollMax  OutDataTypeStr=boolean
  maxq2 : simulink/Logic and Bit Operations/Compare To Constant  relop=<=  const=Estimator.pos.ofPQHovMax  OutDataTypeStr=boolean
  maxw1 : simulink/Logic and Bit Operations/Compare To Constant  relop=<=  const=Estimator.pos.ofPQMax  OutDataTypeStr=boolean
  maxw2 : simulink/Logic and Bit Operations/Compare To Constant  relop=<=  const=Estimator.pos.ofPQMax  OutDataTypeStr=boolean
  maxw3 : simulink/Logic and Bit Operations/Compare To Constant  relop=<=  const=Estimator.pos.deltaDXYMax  OutDataTypeStr=boolean
  maxw4 : simulink/Logic and Bit Operations/Compare To Constant  relop=<=  const=Estimator.pos.deltaDXYMax  OutDataTypeStr=boolean
  minHeightforOF : simulink/Logic and Bit Operations/Compare To Constant  relop=<=  const=Estimator.pos.opticalFlowZMax  OutDataTypeStr=boolean
  enable_flag : Outport  VectorParamsAs1DForOutWhenUnconnected=off
  wires:
  minHeightforOF/1 -> Logical Operator3/4
  IIRgyroz/1 -> DiscreteDerivative/1
  Mux5/1 -> Demux1/1, IIRgyroz/1, Demux4/1
  maxw4/1 -> Logical Operator3/3
  maxw3/1 -> Logical Operator3/2
  dxyOF_datin/1 -> Add/1
  Demux3/2 -> Abs9/1
  Demux3/1 -> Abs8/1
  dxy_estimin/1 -> Add/2
  Add/1 -> Demux3/1
  Abs9/1 -> maxw4/1
  Abs8/1 -> maxw3/1
  Logical Operator2/1 -> Logical Operator3/1
  Logical Operator3/1 -> enable_flag/1
  DiscreteDerivative/1 -> Demux2/1  "dpq"
  Demux2/2 -> Abs7/1
  Demux2/1 -> Abs6/1
  Abs7/1 -> maxdw2/1
  Abs6/1 -> maxdw1/1
  Logical Operator1/1 -> Logical Operator2/2
  Demux1/2 -> Abs5/1
  Demux1/1 -> Abs4/1
  Abs5/1 -> maxq2/1
  Abs4/1 -> maxp2/1
  Abs3/1 -> maxq/1
  Abs2/1 -> maxp/1
  Demux4/2 -> Abs1/1
  Demux4/1 -> Abs/1
  Abs1/1 -> maxw2/1
  Abs/1 -> maxw1/1
  Z_estimin/1 -> minHeightforOF/1
  Logical Operator/1 -> Logical Operator2/1
  maxw1/1 -> Logical Operator/3
  Bus Selector/1 -> Mux5/1  "<p>"
  Selectpitchroll/1 -> Demux5/1
  sensorIMU_datin/1 -> Bus Selector/1
  maxq2/1 -> Logical Operator1/2
  Bus Selector/2 -> Mux5/2  "<q>"
  maxp/1 -> Logical Operator/1
  maxw2/1 -> Logical Operator/4
  orient_estimin/1 -> Selectpitchroll/1
  maxdw1/1 -> Logical Operator/5
  maxdw2/1 -> Logical Operator/6
  maxq/1 -> Logical Operator/2
  Demux5/1 -> Abs2/1
  Demux5/2 -> Abs3/1
  maxp2/1 -> Logical Operator1/1

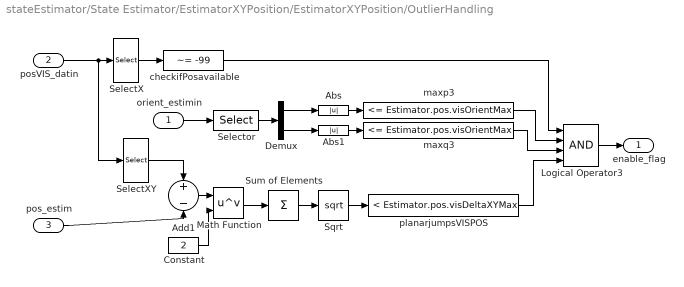
== system stateEstimator/State Estimator/EstimatorXYPosition/EstimatorXYPosition/OutlierHandling ==
  orient_estimin : Inport
  posVIS_datin : Inport  Port=2
  pos_estim : Inport  Port=3
  Abs : Abs
  Abs1 : Abs
  Add1 : Sum  Inputs=+-  AccumDataTypeStr=single
  Constant : Constant  Value=2  OutDataTypeStr=single
  Demux : Demux  Outputs=2
  Logical Operator3 : Logic  Inputs=4  AllPortsSameDT=off  OutDataTypeStr=boolean
  Math Function : Math  Operator=pow  SignedPower=on  SaturateOnIntegerOverflow=on
  SelectX : Selector  InputPortWidth=4  IndexOptions=Index vector (dialog)  Indices=[1]  OutputSizes=1
  SelectXY : Selector  InputPortWidth=4  IndexOptions=Index vector (dialog)  Indices=[1 2]  OutputSizes=1
  Selector : Selector  InputPortWidth=3  IndexOptions=Index vector (dialog)  Indices=[2 3]  OutputSizes=1
  Sqrt : Sqrt  SaturateOnIntegerOverflow=on
  Sum of Elements : Sum  Inputs=+
  checkifPosavailable : simulink/Logic and Bit Operations/Compare To Constant  relop=~=  const=-99  OutDataTypeStr=boolean
  maxp3 : simulink/Logic and Bit Operations/Compare To Constant  relop=<=  const=Estimator.pos.visOrientMax  OutDataTypeStr=boolean
  maxq3 : simulink/Logic and Bit Operations/Compare To Constant  relop=<=  const=Estimator.pos.visOrientMax  OutDataTypeStr=boolean
  planarjumpsVISPOS : simulink/Logic and Bit Operations/Compare To Constant  relop=<  const=Estimator.pos.visDeltaXYMax  OutDataTypeStr=boolean
  enable_flag : Outport  VectorParamsAs1DForOutWhenUnconnected=off
  wires:
  Abs1/1 -> maxq3/1
  Abs/1 -> maxp3/1
  Demux/2 -> Abs1/1
  Demux/1 -> Abs/1
  Selector/1 -> Demux/1
  orient_estimin/1 -> Selector/1
  planarjumpsVISPOS/1 -> Logical Operator3/4
  Sqrt/1 -> planarjumpsVISPOS/1
  pos_estim/1 -> Add1/2
  Add1/1 -> Math Function/1
  SelectXY/1 -> Add1/1
  maxq3/1 -> Logical Operator3/3
  maxp3/1 -> Logical Operator3/2
  Logical Operator3/1 -> enable_flag/1
  checkifPosavailable/1 -> Logical Operator3/1
  SelectX/1 -> checkifPosavailable/1
  posVIS_datin/1 -> SelectX/1, SelectXY/1
  Sum of Elements/1 -> Sqrt/1
  Constant/1 -> Math Function/2
  Math Function/1 -> Sum of Elements/1
